simulink model "edPlane"  (R2023a)
settings: Solver=VariableStepAuto  StartTime=0.0  StopTime=5  RelTol=1e-3
values from neighbouring files (symbols this model uses):
  Alon = [Xu Xw 0 -g*cos(theta0);         Zu Zw u0 -g*sin(theta0);         Mu Mw Mq        0;         0  0  1         0]    [plane_init.m]
  Blon = [Xdele XdelT;         Zdele ZdelT;         Mdele MdelT;         0       0]    [plane_init.m]
  w_e = 30    [plane_init.m]
  w_t = 2    [plane_init.m]
  zeta_e = 0.7    [plane_init.m]
  zeta_t = 1.1    [plane_init.m]
libraries: simulink_extras x2
settings Model: Creator=eduar  LastModifiedBy=eduar
settings OptimizationCC: ReuseModelBlockBuffer=off

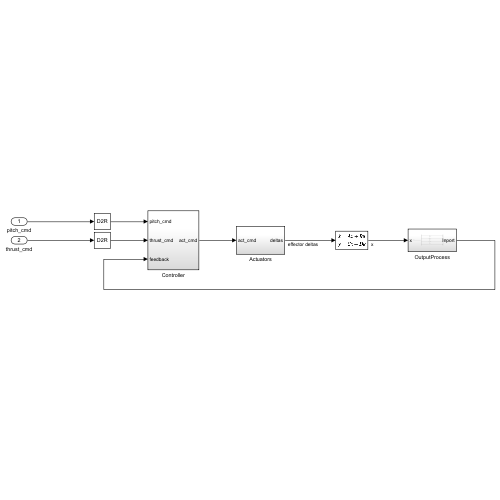
[thumbnail: Simulink's stored preview of the top-level diagram]
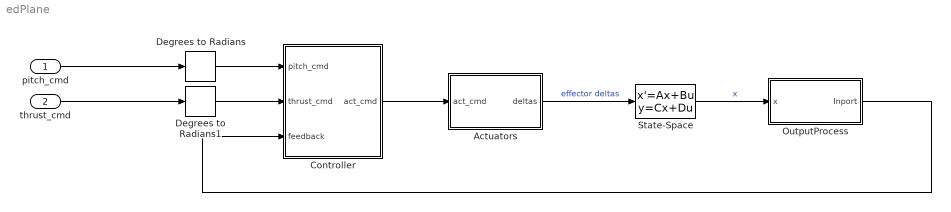
== system edPlane ==
  pitch_cmd : Inport
  thrust_cmd : Inport  Port=2
  Actuators : Subsystem
  Controller : Subsystem
  Degrees to Radians : simulink_extras/Transformations/Degrees to Radians
  Degrees to Radians1 : simulink_extras/Transformations/Degrees to Radians
  OutputProcess : Subsystem
  State-Space : StateSpace  A=Alon  B=Blon  C=[1 0 0 0; 0 1 0 0; 0 0 1 0; 0 0 0 1]  D=[0 0; 0 0 ; 0 0; 0 0]  InitialCondition=0
  wires:
  State-Space/1 -> OutputProcess/1(x)  "x"
  OutputProcess/1(Inport) -> Controller/3(feedback)
  Actuators/1(deltas) -> State-Space/1  "effector deltas"
  Controller/1(act_cmd) -> Actuators/1(act_cmd)
  Degrees to Radians/1 -> Controller/1(pitch_cmd)
  Degrees to Radians1/1 -> Controller/2(thrust_cmd)
  pitch_cmd/1 -> Degrees to Radians/1
  thrust_cmd/1 -> Degrees to Radians1/1

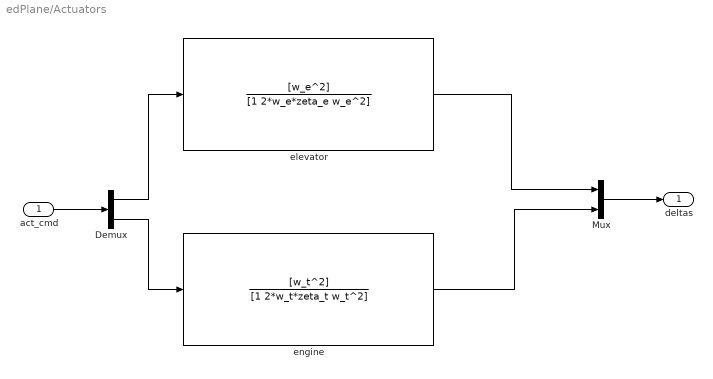
== system edPlane/Actuators ==
  act_cmd : Inport
  Demux : Demux  Outputs=2
  Mux : Mux  Inputs=2
  elevator : TransferFcn  Numerator=[w_e^2]  Denominator=[1 2*w_e*zeta_e w_e^2]
  engine : TransferFcn  Numerator=[w_t^2]  Denominator=[1 2*w_t*zeta_t w_t^2]
  deltas : Outport
  wires:
  act_cmd/1 -> Demux/1
  Demux/1 -> elevator/1
  Mux/1 -> deltas/1
  Demux/2 -> engine/1
  elevator/1 -> Mux/1
  engine/1 -> Mux/2

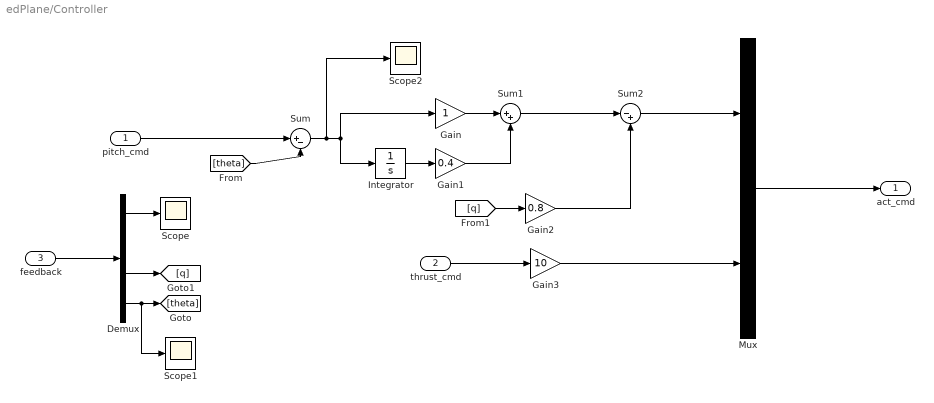
== system edPlane/Controller ==
  pitch_cmd : Inport
  thrust_cmd : Inport  Port=2
  feedback : Inport  Port=3
  Demux : Demux
  Gain : Gain
  Gain1 : Gain  Gain=0.4
  Gain2 : Gain  Gain=0.8
  Gain3 : Gain  Gain=10
  Integrator : Integrator
  Mux : Mux  Inputs=2
  Scope : Scope
  Scope1 : Scope
  Scope2 : Scope
  Sum : Sum  Inputs=|+-
  Sum1 : Sum  Inputs=|++
  Sum2 : Sum  Inputs=|-+
  act_cmd : Outport
  wires:
  Mux/1 -> act_cmd/1
  feedback/1 -> Demux/1
  pitch_cmd/1 -> Sum/1
  Sum/1 -> Scope2/1, Gain/1, Integrator/1
  Demux/4 -> Scope1/1, [theta]
  [theta] -> Sum/2
  Integrator/1 -> Gain1/1
  Gain/1 -> Sum1/1
  Gain1/1 -> Sum1/2
  Sum1/1 -> Sum2/1
  Demux/3 -> [q]
  [q] -> Gain2/1
  Gain2/1 -> Sum2/2
  thrust_cmd/1 -> Gain3/1
  Demux/1 -> Scope/1
  Sum2/1 -> Mux/1
  Gain3/1 -> Mux/2

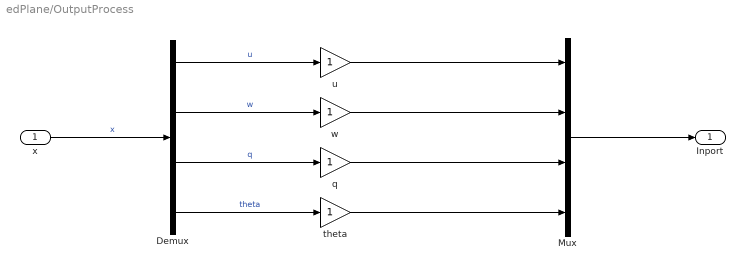
== system edPlane/OutputProcess ==
  x : Inport
  Demux : Demux
  Mux : Mux
  q : Gain
  theta : Gain
  u : Gain
  w : Gain
  Inport : Outport
  wires:
  x/1 -> Demux/1  "x"
  Demux/1 -> u/1  "u"
  u/1 -> Mux/1
  Demux/2 -> w/1  "w"
  Demux/3 -> q/1  "q"
  Demux/4 -> theta/1  "theta"
  w/1 -> Mux/2
  q/1 -> Mux/3
  theta/1 -> Mux/4
  Mux/1 -> Inport/1
